simulink model "Tutorial6_RaspberryPiAct_2dot017_final"  (R2025b)
settings: Solver=FixedStepAuto  StartTime=0.0  StopTime=90  FixedStep=0.1  RelTol=1e-3  EnableMultiTasking=on
undefined symbols (not defined in the file): Green, led0
libraries: raspberrypiBasiclib x5
settings Model: ExtModeTrigDuration=2  Creator=david  LastModifiedBy=david
settings SolverCC: PositivePriorityOrder=on  AutoInsertRateTranBlk=on
settings DataIOCC: SaveOutput=off  DSMLogging=off  SaveTime=off  ReturnWorkspaceOutputs=off
settings OptimizationCC: EnhancedBackFolding=on  PassReuseOutputArgsAs=Individual arguments  ZeroExternalMemoryAtStartup=off  ZeroInternalMemoryAtStartup=off  MaxStackSize=200000  OptimizeBlockOrder=speed  DifferentSizesBufferReuse=on  OptimizationCustomize=off  EfficientTunableParamExpr=on
settings DebuggingCC: ParameterTunabilityLossMsg=error
settings HardwareCC: ProdBitPerPointer=32.0  ProdBitPerSizeT=32.0  ProdBitPerPtrDiffT=32.0  ProdLargestAtomicInteger=Long  ProdLargestAtomicFloat=Double  ProdWordSize=32.0  ProdLongLongMode=on  ProdHWDeviceType=ARM Compatible->ARM Cortex-A (32-bit)
settings RTWCC: SystemTargetFile=ert.tlc  HardwareBoard=Raspberry Pi  TLCOptions="-aInlineSetEventsForThisBaseRateFcn=TLC_FALSE -aSuppressMultiTaskScheduler=TLC_FALSE  -aRateBasedStepFcn=0"  TemplateMakefile=ert_default_tmf  Toolchain=GNU GCC Embedded Linux  BuildConfiguration=Faster Runs  CheckMdlBeforeBuild=Warning  Description=Embedded Coder
settings CodeAppCC: ForceParamTrailComments=on  IgnoreCustomStorageClasses=off  OperatorAnnotations=on  SimulinkDataObjDesc=on  SFDataObjDesc=on  InsertBlockDesc=on
settings ERTTargetCC: ExtModeTransport=2.0  ExtModeStaticAlloc=on  ExtModeMexFile=ext_xcp  ExtModeIntrfLevel=Level2 - Open  InlinedParameterPlacement=Hierarchical  CodeReplacementLibrary=ARM Cortex-A CMSIS  SupportContinuousTime=on  SupportVariableSizeSignals=on

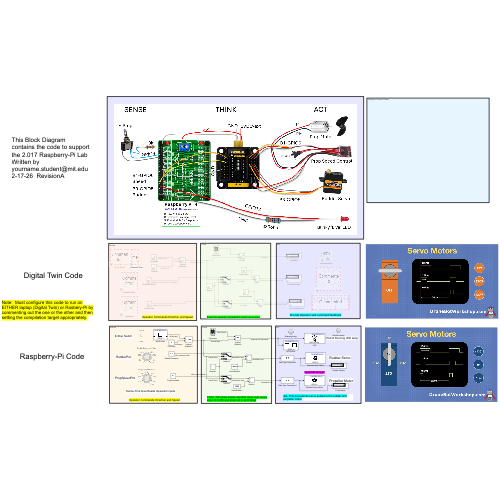
[thumbnail: Simulink's stored preview of the top-level diagram]
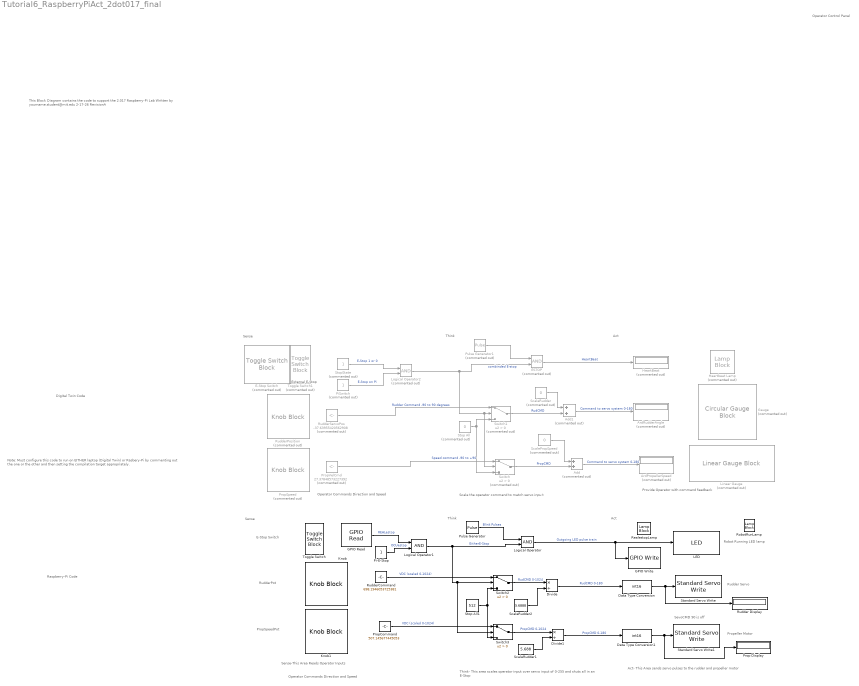
== system Tutorial6_RaspberryPiAct_2dot017_final ==
  note: Operator Control Panel
  note: External E-Stop
  note: SevoCMD 90 is off
  note: Provide Operator with command feedback
  note: Scale the operator command to match servo inpu t
  note: Operator Commands Direction and Speed
  note: Act- This Area sends servo pulses to the rudder and propeller motor
  note: Think- This area scales operator input over servo input of 0-255 and shuts all in an E-Stop
  note: Sense-This Area Reads Operator Inputs
  note: Rudder Servo
  note: Robot Running LED lamp
  note: Note: Must configure this code to run on EITHER laptop (Digital Twin) or Rasbery-Pi by commenting out the one or the other and then setting the compilation target appropriately.
  note: Digital Twin Code
  note: E-Stop Switch
  note: RudderPot
  note: Act
  note: Think
  note: Sense
  note: This Block Diagram contains the code to support the 2.017 Raspberry-Pi Lab
      | Written by yourname.student@mit.edu 2-17-26 RevisionA
  note: Sense
  note: Act
  note: Think
  note: Raspberry-Pi Code
  note: Operator Commands Direction and Speed
  note: PropSpeedPot
  note: Propeller Motor
  Add : Sum  Commented=on
  Add1 : Sum  Commented=on
  ArdPropellerSpeed : Display  Commented=on
  ArdRudderAngle : Display  Commented=on
  Data Type Conversion : DataTypeConversion  OutMin=0  OutMax=180  OutDataTypeStr=int16  SaturateOnIntegerOverflow=off  RndMeth=Floor
  Data Type Conversion1 : DataTypeConversion  OutMin=0  OutMax=180  OutDataTypeStr=int16  SaturateOnIntegerOverflow=off  RndMeth=Floor
  Divide : Product  Inputs=*/
  Divide1 : Product  Inputs=*/
  E-Stop Switch : ToggleSwitchBlock  Commented=on
  ESTOP : Logic  Commented=on  AllPortsSameDT=off  OutDataTypeStr=boolean
  GPIO Read : raspberrypiBasiclib/GPIO Read  BoardProperty=Pi 4 Model B  gpio=4  SampleTime=-1  blockPlatform=Raspberry Pi  PinNumber=4  board=[]  direction=[]  internalResistor=[]
  GPIO Write : raspberrypiBasiclib/GPIO Write  BoardProperty=Pi 4 Model B  gpio=13  blockPlatform=Raspberry Pi  PinNumber=17  board=[]  direction=[]
  Gauge : CircularGaugeBlock  Commented=on  ScaleMin=-100  FontColor=[0.0, 0.0, 0.0]
  HeartBeat : Display  Commented=on
  Heartbeat Lamp : LampBlock  Commented=on  LabelPosition=Hide  DefaultColor=[192.0, 192.0, 192.0]
  Knob : KnobBlock  ScaleMax=1024
  Knob1 : KnobBlock  ScaleMax=1024
  LED : raspberrypiBasiclib/LED  BoardProperty=Pi 5 Model  LED_=led0 (Green)
  Linear Gauge : LinearGaugeBlock  Commented=on  ScaleMin=-100  FontColor=[0.0, 0.0, 0.0]
  Logical Operator : Logic  AllPortsSameDT=off  OutDataTypeStr=boolean
  Logical Operator1 : Logic  AllPortsSameDT=off  OutDataTypeStr=Inherit: Inherit via back propagation
  Logical Operator2 : Logic  Commented=on  AllPortsSameDT=off  OutDataTypeStr=boolean
  Pi-E-Stop : Constant  OutDataTypeStr=Inherit: Inherit via back propagation
  PiSwitch : Constant  Commented=on
  Prop Display : Display
  PropCommand : Constant  Value=507.145677445053
  PropSpeed : KnobBlock  Commented=on  ScaleMin=-90  ScaleMax=90
  PropVelCmd : Constant  Commented=on  Value=27.37848573227392
  Pulse Generator : DiscretePulseGenerator  PulseType=Time based  PulseWidth=50
  Pulse Generator1 : DiscretePulseGenerator  Commented=on  PulseType=Time based  Period=4  PulseWidth=50
  RealestopLamp : LampBlock  LabelPosition=Hide  DefaultColor=[192.0, 192.0, 192.0]
  RobotRunLamp : LampBlock  LabelPosition=Hide  DefaultColor=[192.0, 192.0, 192.0]
  Rudder Display : Display
  RudderCommand : Constant  Value=698.1946053725381
  RudderPosition : KnobBlock  Commented=on  ScaleMin=-90  ScaleMax=90
  RudderServoPos : Constant  Commented=on  Value=-37.63955420562908
  ScalePropSpeed : Constant  Commented=on  Value=0
  ScaleRudder : Constant  Commented=on  Value=0
  ScaleRudder1 : Constant  Value=5.688
  ScaleRudder2 : Constant  Value=5.6888
  Standard Servo Write : raspberrypiBasiclib/Standard Servo Write  board=Pi 4 Model B  Pin_=5  MinPulseDuration=700e-6  MaxPulseDuration=2000e-6  blockPlatform=Raspberry Pi
  Standard Servo Write1 : raspberrypiBasiclib/Standard Servo Write  board=Pi 4 Model B  Pin_=6  MinPulseDuration=700e-6  MaxPulseDuration=2000e-6  blockPlatform=Raspberry Pi
  Stop All : Constant  Commented=on  Value=0
  Stop All1 : Constant  Value=512
  StopState : Constant  Commented=on
  Switch : Switch  Commented=on  Criteria=u2 > Threshold  SaturateOnIntegerOverflow=off  InputSameDT=off
  Switch1 : Switch  Commented=on  Criteria=u2 > Threshold  SaturateOnIntegerOverflow=off  InputSameDT=off
  Switch2 : Switch  Criteria=u2 > Threshold  SaturateOnIntegerOverflow=off  InputSameDT=off
  Switch3 : Switch  Criteria=u2 > Threshold  SaturateOnIntegerOverflow=off  InputSameDT=off
  Toggle Switch : ToggleSwitchBlock  LabelPosition=Hide
  Toggle Switch1 : ToggleSwitchBlock  Commented=on
  wires:
  Pulse Generator/1 -> Logical Operator/1  "Blink Pulses"
  Logical Operator/1 -> GPIO Write/1, LED/1  "Outgoing LED pulse train"
  Pulse Generator1/1 -> ESTOP/1
  ESTOP/1 -> HeartBeat/1  "HeartBeat"
  ScaleRudder/1 -> Add1/1
  ScalePropSpeed/1 -> Add/1
  RudderServoPos/1 -> Switch1/1  "Rudder Command -90 to 90 degrees"
  Stop All/1 -> Switch/3, Switch1/3
  PropVelCmd/1 -> Switch/1  "Speed command -90 to +90"
  Switch1/1 -> Add1/2  "RudCMD"
  Switch/1 -> Add/2  "PropCMD"
  Add1/1 -> ArdRudderAngle/1  "Command to servo system 0-180"
  Add/1 -> ArdPropellerSpeed/1  "Command to servo system 0-180"
  RudderCommand/1 -> Switch2/1  "VDC (scaled 0-1024)"
  PropCommand/1 -> Switch3/1  "VDC (scaled 0-1024)"
  Stop All1/1 -> Switch2/3, Switch3/3
  Switch3/1 -> Divide1/1  "PropCMD 0-1024"
  Switch2/1 -> Divide/1  "RudCMD 0-1024"
  ScaleRudder2/1 -> Divide/2
  Divide/1 -> Data Type Conversion/1  "RudCMD 0-180"
  ScaleRudder1/1 -> Divide1/2
  Divide1/1 -> Data Type Conversion1/1  "PropCMD 0-180"
  Data Type Conversion/1 -> Rudder Display/1, Standard Servo Write/1
  Data Type Conversion1/1 -> Prop Display/1, Standard Servo Write1/1
  Logical Operator1/1 -> Switch3/2, Switch2/2, Logical Operator/2  "EitherE-Stop"
  Pi-E-Stop/1 -> Logical Operator1/2  "OCUestop"
  GPIO Read/1 -> Logical Operator1/1  "REALestop"
  Logical Operator2/1 -> Switch/2, Switch1/2, ESTOP/2  "combinded E-stop"
  StopState/1 -> Logical Operator2/1  "E-Stop 1 or 0"
  PiSwitch/1 -> Logical Operator2/2  "E-Stop on Pi"
